simulink model "filter8tap"  (Simulink 7.1)
settings: Solver=ode45  StartTime=0.0  StopTime=100.0  RelTol=1e-3
InitFcn:
  | %% DSPBuilder Start
  | alt_dspbuilder_update_model(bdroot)
  | %% DSPBuilder End
libraries: allblocks_alteradspbuilder2 x10
settings Model: Creator=gnixon  LastModifiedBy=delphick
settings DataIOCC: SignalLoggingName=sigsOut
settings DebuggingCC: SaveWithParameterizedLinksMsg=none  SignalResolutionControl=TryResolveAllWithWarning  SolverPrmCheckMsg=none  MultiTaskDSMMsg=warning  MultiTaskCondExecSysMsg=none  UnconnectedOutputMsg=none
settings HardwareCC: TargetUnknown=on
settings RTWCC: IncludeERTFirstTime=on
settings GRTTargetCC: TargetFcnLib=ansi_tfl_tmw.mat  ModelReferenceCompliant=off  MatFileLogging=off

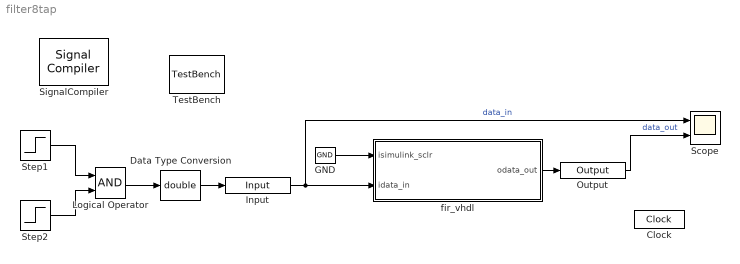
== system filter8tap ==
  Clock : allblocks_alteradspbuilder2/Clock  ClockPeriod=20  ClockPeriodUnit=ns  SampleTime=1  ResetLatency=0  ResetRegisterCascadeDepth=0  SimulationStartCycle=5  PhaseOffset=0  Reset=aclr  ResetType=Active High  Export=off
  Data Type Conversion : DataTypeConversion  OutDataTypeMode=double  OutDataType=sfix(16)  OutScaling=2^0  OutDataTypeStr=double  SaturateOnIntegerOverflow=on  RndMeth=Zero
  GND : allblocks_alteradspbuilder2/GND  SpecifyClock=off
  Input : allblocks_alteradspbuilder2/Input  iofile=D:\temp\DSPBuilderTEST\BasicLibraryTests_AltLab_BlackBox_SysWithReset_filter8tap.mdl\tb_filter8tap\filter8tap_Input.salt  BusType=Signed Integer  bwl=16  bwr=0  SpecifyClock=off  PORTTYPE=Input  externalType=Inferred  allowFloatingPointOverride=on  logOutputs=off
  Logical Operator : Logic  AllPortsSameDT=off
  Output : allblocks_alteradspbuilder2/Output  iofile=D:\temp\DSPBuilderTEST\BasicLibraryTests_AltLab_BlackBox_SysWithReset_filter8tap.mdl\tb_filter8tap\filter8tap_Output.capture  BusType=Signed Integer  bwl=33  bwr=0  externalType=Inferred  PORTTYPE=Output  allowFloatingPointOverride=on  logOutputs=off
  Scope : Scope  NumInputPorts=2
      settings: YMin=-5~-5  YMax=5~5
  SignalCompiler : allblocks_alteradspbuilder2/Signal Compiler  DeviceFamily=Stratix III  DeviceName=AUTO  EnableSignalTap=off  SignalTapDepth=128  UseBoardBlock=off  StpUseDefaultClock=on  StpClock=Clock  ExportDir=.
  Step1 : Step  Time=10  SampleTime=1
  Step2 : Step  Time=11  Before=1  After=0  SampleTime=1
  TestBench : allblocks_alteradspbuilder2/TestBench  enable=on  advancedMode=off  modelSimGui=off  maxDisplayErrors=10  mismatchErrorLevel=Error  simdatafile=D:\temp\DSPBuilderTEST\BasicLibraryTests_AltLab_BlackBox_SysWithReset_filter8tap.mdl\tb_filter8tap\filter8tap.simdata.tcl
  fir_vhdl : Subsystem
      mask Type: SubSystem AlteraBlockSet
  wires:
  Step1/1 -> Logical Operator/1
  Step2/1 -> Logical Operator/2
  Logical Operator/1 -> Data Type Conversion/1
  GND/1 -> fir_vhdl/1(isimulink_sclr)
  Input/1 -> Scope/1, fir_vhdl/2(idata_in)  "data_in"
  fir_vhdl/1(odata_out) -> Output/1
  Output/1 -> Scope/2  "data_out"
  Data Type Conversion/1 -> Input/1

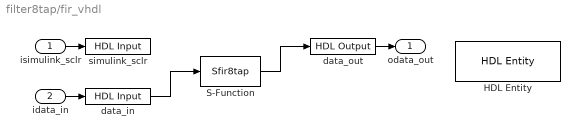
== system filter8tap/fir_vhdl ==
  isimulink_sclr : Inport  OutDataType=sfix(16)  OutScaling=2^0
  idata_in : Inport  Port=2  OutDataType=sfix(16)  OutScaling=2^0
  HDL Entity : allblocks_alteradspbuilder2/HDL Entity  HDLFile=fir_vhdl.vhd  clockname=simulink_clock  resetname=simulink_sclr  useSubsystemPortName=off
  S-Function : S-Function  FunctionName=Sfir8tap  Parameters=-1 3962 4817 5420 5733 5733 5420 4817 3962  EnableBusSupport=off
  data_in : allblocks_alteradspbuilder2/HDL Input  BusType=Signed Integer  bwl=16  bwr=0  externalType=Inferred
  data_out : allblocks_alteradspbuilder2/HDL Output  BusType=Signed Integer  bwl=33  bwr=0  externalType=Inferred
  simulink_sclr : allblocks_alteradspbuilder2/HDL Input  BusType=Single Bit  bwl=1  bwr=0  externalType=Inferred
  odata_out : Outport  OutDataType=sfix(16)  OutScaling=2^0
  wires:
  isimulink_sclr/1 -> simulink_sclr/1
  idata_in/1 -> data_in/1
  data_out/1 -> odata_out/1
  data_in/1 -> S-Function/1
  S-Function/1 -> data_out/1
